simulink model "test"  (R2024b)
settings: Solver=ode4  StartTime=t0  StopTime=tf  FixedStep=0.01  RelTol=1e-3
settings Model: Creator=esteb  LastModifiedBy=esteb

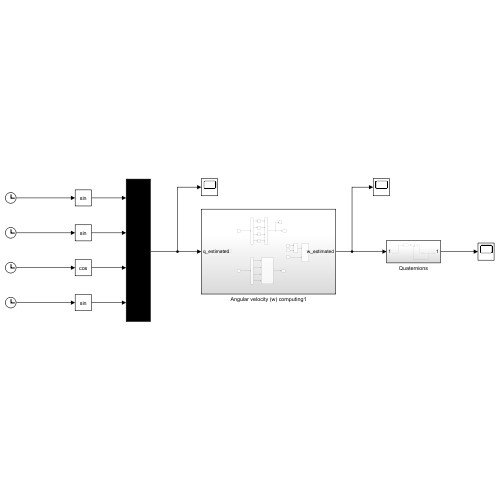
[thumbnail: Simulink's stored preview of the top-level diagram]
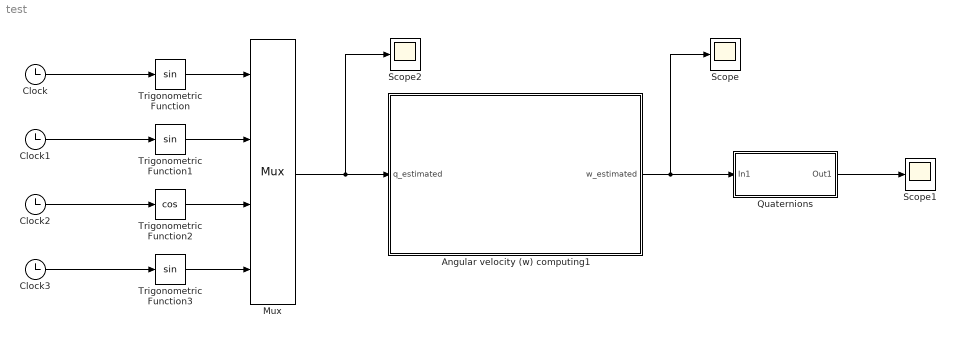
== system test ==
  Angular velocity (w) computing1 : Subsystem
  Clock{,1..3} (4 alike) : Clock
  Mux : Mux
  Quaternions : Subsystem
  Scope : Scope
  Scope1 : Scope
  Scope2 : Scope
  Trigonometric Function : Trigonometry
  Trigonometric Function1 : Trigonometry
  Trigonometric Function2 : Trigonometry  Operator=cos
  Trigonometric Function3 : Trigonometry
  wires:
  Angular velocity (w) computing1/1(w_estimated) -> Scope/1, Quaternions/1(In1)
  Quaternions/1(Out1) -> Scope1/1
  Mux/1 -> Scope2/1, Angular velocity (w) computing1/1(q_estimated)
  Trigonometric Function/1 -> Mux/1
  Clock/1 -> Trigonometric Function/1
  Clock3/1 -> Trigonometric Function3/1
  Trigonometric Function3/1 -> Mux/4
  Clock2/1 -> Trigonometric Function2/1
  Trigonometric Function2/1 -> Mux/3
  Clock1/1 -> Trigonometric Function1/1
  Trigonometric Function1/1 -> Mux/2

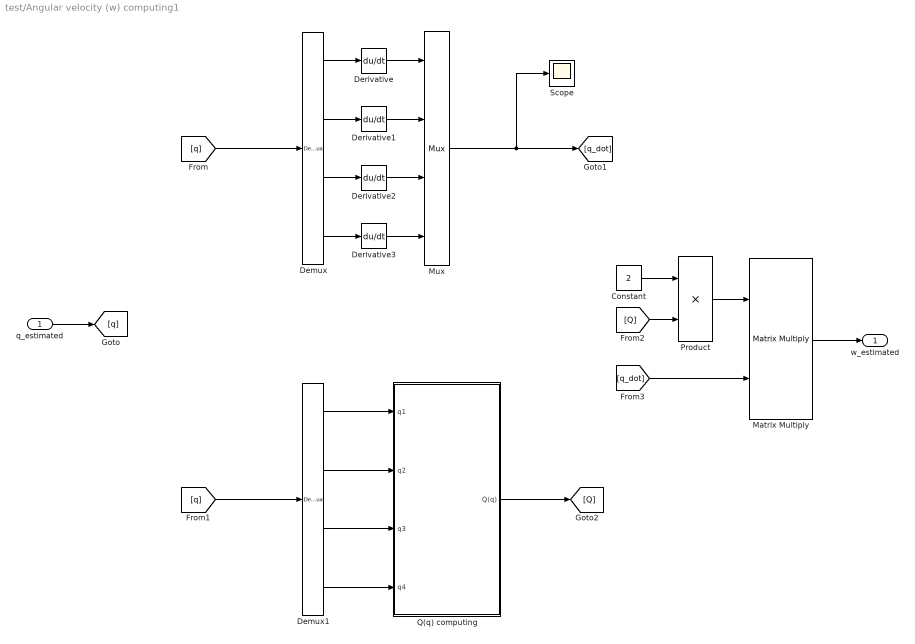
== system test/Angular velocity (w) computing1 ==
  q_estimated : Inport
  Constant : Constant  Value=2
  Demux : Demux
  Demux1 : Demux
  Derivative{,1..3} (4 alike) : Derivative
  Matrix Multiply : Product  Multiplication=Matrix(*)
  Mux : Mux
  Product : Product
  Q(q) computing : Subsystem
  Scope : Scope
  w_estimated : Outport
  wires:
  q_estimated/1 -> [q]
  [q] -> Demux/1
  Demux/1 -> Derivative/1
  Demux/2 -> Derivative1/1
  Demux/3 -> Derivative2/1
  Demux/4 -> Derivative3/1
  [q] -> Demux1/1
  Demux1/1 -> Q(q) computing/1(q1)
  Demux1/4 -> Q(q) computing/4(q4)
  Demux1/3 -> Q(q) computing/3(q3)
  Demux1/2 -> Q(q) computing/2(q2)
  Mux/1 -> [q_dot], Scope/1
  Q(q) computing/1(Q(q)) -> [Q]
  [Q] -> Product/2
  Constant/1 -> Product/1
  [q_dot] -> Matrix Multiply/2
  Matrix Multiply/1 -> w_estimated/1
  Derivative/1 -> Mux/1
  Derivative1/1 -> Mux/2
  Derivative2/1 -> Mux/3
  Derivative3/1 -> Mux/4
  Product/1 -> Matrix Multiply/1

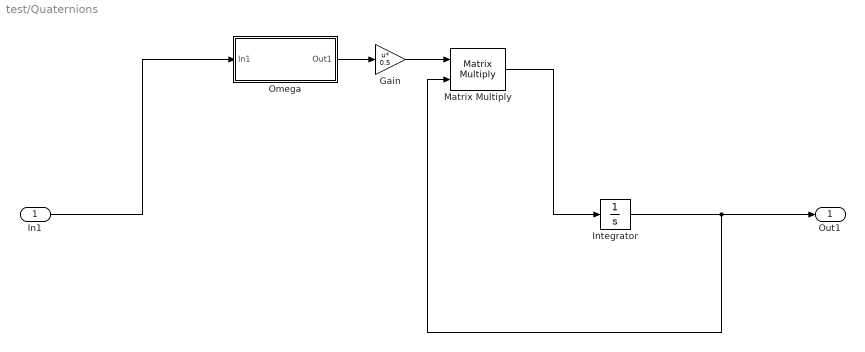
== system test/Quaternions ==
  In1 : Inport
  Gain : Gain  Gain=0.5  Multiplication=Matrix(u*K)
  Integrator : Integrator  InitialCondition=[0; 1; 1; 0]
  Matrix Multiply : Product  Multiplication=Matrix(*)
  Omega : Subsystem
  Out1 : Outport
  wires:
  Integrator/1 -> Matrix Multiply/2, Out1/1
  In1/1 -> Omega/1(In1)
  Omega/1(Out1) -> Gain/1
  Gain/1 -> Matrix Multiply/1
  Matrix Multiply/1 -> Integrator/1

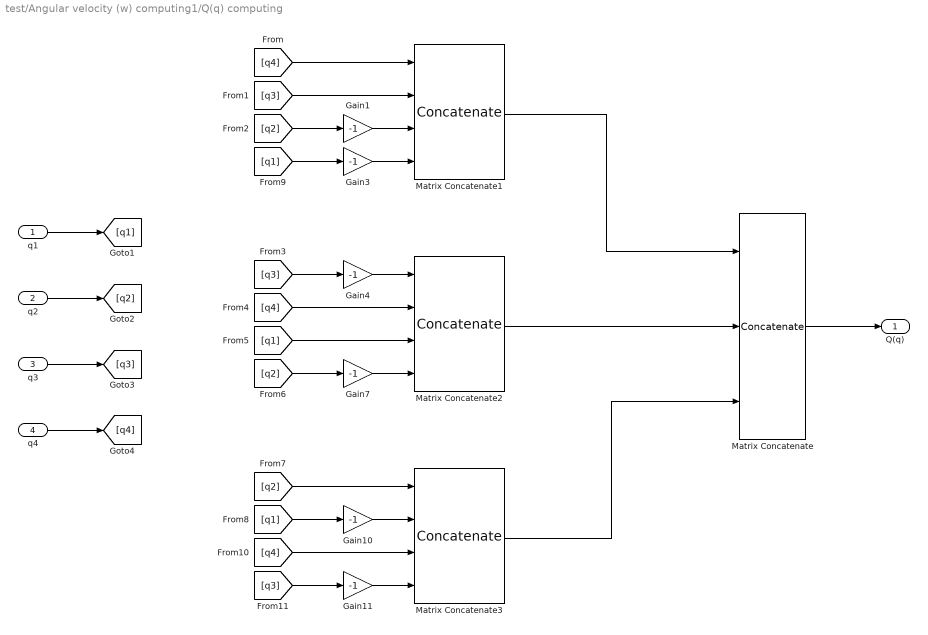
== system test/Angular velocity (w) computing1/Q(q) computing ==
  q1 : Inport
  q2 : Inport  Port=2
  q3 : Inport  Port=3
  q4 : Inport  Port=4
  Gain{1,3..4,7,10..11} (6 alike) : Gain  Gain=-1
  Matrix Concatenate : Concatenate  NumInputs=3  Mode=Multidimensional array
  Matrix Concatenate1 : Concatenate  NumInputs=4  Mode=Multidimensional array  ConcatenateDimension=2
  Matrix Concatenate2 : Concatenate  NumInputs=4  Mode=Multidimensional array  ConcatenateDimension=2
  Matrix Concatenate3 : Concatenate  NumInputs=4  Mode=Multidimensional array  ConcatenateDimension=2
  Q(q) : Outport
  wires:
  q1/1 -> [q1]
  q2/1 -> [q2]
  q3/1 -> [q3]
  q4/1 -> [q4]
  [q4] -> Matrix Concatenate1/1
  [q3] -> Matrix Concatenate1/2
  Gain1/1 -> Matrix Concatenate1/3
  [q2] -> Gain1/1
  Matrix Concatenate1/1 -> Matrix Concatenate/1
  Matrix Concatenate/1 -> Q(q)/1
  [q1] -> Gain3/1
  Gain3/1 -> Matrix Concatenate1/4
  [q2] -> Gain7/1
  [q1] -> Matrix Concatenate2/3
  Gain7/1 -> Matrix Concatenate2/4
  [q3] -> Gain4/1
  [q4] -> Matrix Concatenate2/2
  Gain4/1 -> Matrix Concatenate2/1
  [q3] -> Gain11/1
  [q4] -> Matrix Concatenate3/3
  [q1] -> Gain10/1
  Gain11/1 -> Matrix Concatenate3/4
  Gain10/1 -> Matrix Concatenate3/2
  [q2] -> Matrix Concatenate3/1
  Matrix Concatenate2/1 -> Matrix Concatenate/2
  Matrix Concatenate3/1 -> Matrix Concatenate/3

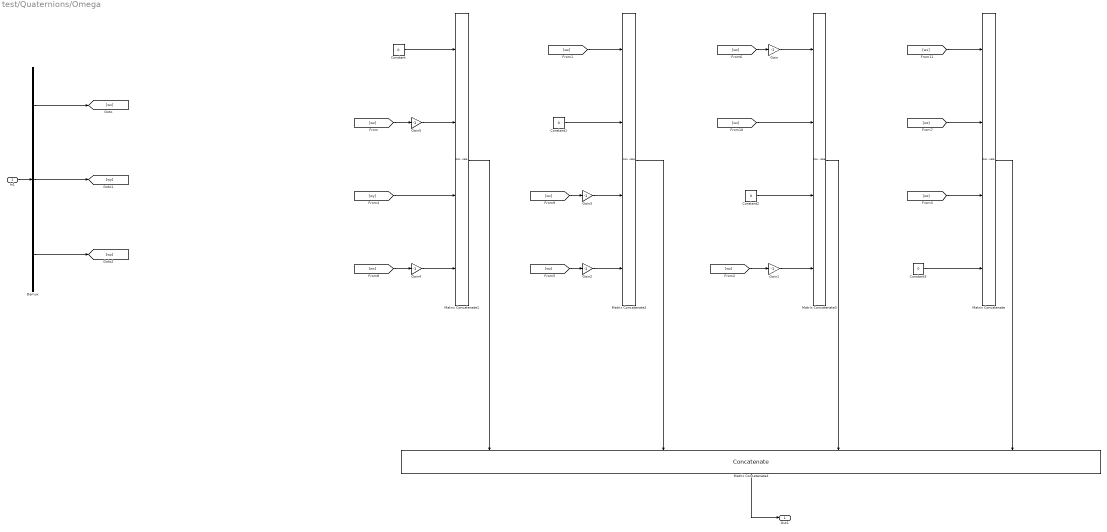
== system test/Quaternions/Omega ==
  In1 : Inport
  Constant{,1..3} (4 alike) : Constant  Value=0
  Demux : Demux  Outputs=3
  Gain{,1..5} (6 alike) : Gain  Gain=-1
  Matrix Concatenate{,1..3} (4 alike) : Concatenate  NumInputs=4  Mode=Multidimensional array
  Matrix Concatenate4 : Concatenate  NumInputs=4  Mode=Multidimensional array  ConcatenateDimension=2
  Out1 : Outport
  wires:
  In1/1 -> Demux/1
  Demux/1 -> [wx]
  Demux/2 -> [wy]
  Demux/3 -> [wz]
  Matrix Concatenate1/1 -> Matrix Concatenate4/1
  Matrix Concatenate2/1 -> Matrix Concatenate4/2
  Matrix Concatenate/1 -> Matrix Concatenate4/4
  Matrix Concatenate3/1 -> Matrix Concatenate4/3
  Constant/1 -> Matrix Concatenate1/1
  Constant1/1 -> Matrix Concatenate2/2
  Constant2/1 -> Matrix Concatenate3/3
  Constant3/1 -> Matrix Concatenate/4
  Gain/1 -> Matrix Concatenate3/1
  Gain1/1 -> Matrix Concatenate3/4
  Gain2/1 -> Matrix Concatenate2/4
  Gain3/1 -> Matrix Concatenate2/3
  Gain4/1 -> Matrix Concatenate1/4
  Gain5/1 -> Matrix Concatenate1/2
  [wz] -> Gain5/1
  [wz] -> Matrix Concatenate2/1
  [wz] -> Gain1/1
  [wz] -> Matrix Concatenate/3
  [wy] -> Matrix Concatenate1/3
  [wz] -> Gain2/1
  [wz] -> Gain/1
  [wz] -> Matrix Concatenate/2
  Matrix Concatenate4/1 -> Out1/1
  [wx] -> Gain4/1
  [wx] -> Gain3/1
  [wx] -> Matrix Concatenate3/2
  [wx] -> Matrix Concatenate/1
